simulink model "c10mimps"  (R2017a)
settings: Solver=ode45  StartTime=0.0  StopTime=10.0  RelTol=1e-10
undefined symbols (not defined in the file): n, ww
libraries: simulink x1
settings Model: Creator=Professor Dingyu Xue  LastModifiedBy=Professor Dingyu Xue
settings DataIOCC: SaveFormat=Array
settings OptimizationCC: LifeSpan=inf
settings DebuggingCC: FcnCallInpInsideContextMsg=warning  SFExecutionAtInitializationDiag=none
settings HardwareCC: ProdBitPerSizeT=32  ProdBitPerPtrDiffT=32  ProdWordSize=32  ProdHWDeviceType=Specified

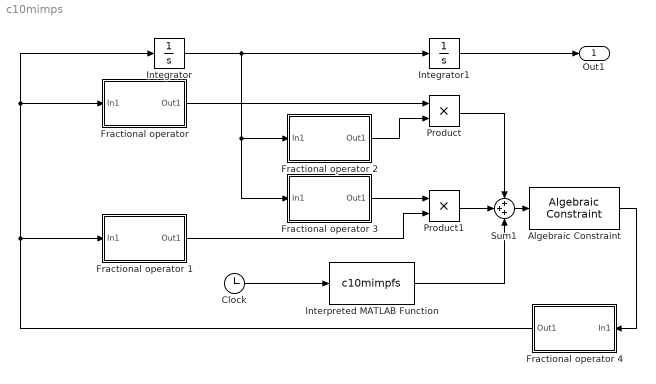
== system c10mimps ==
  Algebraic Constraint : simulink/Math Operations/Algebraic Constraint  z0=0
      settings: SourceProductName=Simulink  SourceProductBaseCode=SL
  Clock : Clock
  "Fractional operator " : Subsystem  mask{gam=-0.2, ww=ww, n=n, kF1=on, kF=Oustaloup filter}
      mask prompts: gam "Derivative order gamma"; ww "Frequency range [wb,wh]"; n "Apprixmation order"; kF1 "Is a low-pass filter required?"; kF "Filter type"
      mask init:
      | wb=ww(1); wh=ww(2); 
      | if kF==1, G=ousta_fod(gam,n,wb,wh);
      | else, G=new_fod(gam,n,wb,wh); end
      | num=G.num{1}; den=G.den{1}; T=1/wh; str='Fractional\n';
      | if isnumeric(gam)
      | 	if gam>0, str=[str, 'Der  s^' num2str(gam) ];
      | 	else, str=[str, 'Int  s^{' num2str(gam) '}']; end
      | else, str=[str, 'Der  s^gam']; end
      | if kF1==1, G=G*tf(1,[T 1]); end
      mask TypeOptions kF: Oustaloup filter | Modified Oustaloup filter
      mask Display: disp(str)
  Fractional operator 1 : Subsystem  mask{gam=-0.3, ww=ww, n=n, kF1=on, kF=Oustaloup filter}
      mask prompts: gam "Derivative order gamma"; ww "Frequency range [wb,wh]"; n "Apprixmation order"; kF1 "Is a low-pass filter required?"; kF "Filter type"
      mask init: same as c10mimps/Fractional operator 
      mask TypeOptions kF: Oustaloup filter | Modified Oustaloup filter
      mask Display: disp(str)
  Fractional operator 2 : Subsystem  mask{gam=-0.8, ww=ww, n=n, kF1=on, kF=Oustaloup filter}
      mask prompts: gam "Derivative order gamma"; ww "Frequency range [wb,wh]"; n "Apprixmation order"; kF1 "Is a low-pass filter required?"; kF "Filter type"
      mask init: same as c10mimps/Fractional operator 
      mask TypeOptions kF: Oustaloup filter | Modified Oustaloup filter
      mask Display: disp(str)
  Fractional operator 3 : Subsystem  mask{gam=-0.7, ww=ww, n=n, kF1=on, kF=Oustaloup filter}
      mask prompts: gam "Derivative order gamma"; ww "Frequency range [wb,wh]"; n "Apprixmation order"; kF1 "Is a low-pass filter required?"; kF "Filter type"
      mask init: same as c10mimps/Fractional operator 
      mask TypeOptions kF: Oustaloup filter | Modified Oustaloup filter
      mask Display: disp(str)
  Fractional operator 4 : Subsystem  mask{gam=0.2, ww=ww, n=n, kF1=on, kF=Oustaloup filter}
      mask prompts: gam "Derivative order gamma"; ww "Frequency range [wb,wh]"; n "Apprixmation order"; kF1 "Is a low-pass filter required?"; kF "Filter type"
      mask init: same as c10mimps/Fractional operator 
      mask TypeOptions kF: Oustaloup filter | Modified Oustaloup filter
      mask Display: disp(str)
  Integrator : Integrator  InitialCondition=-1/2
  Integrator1 : Integrator  InitialCondition=1
  Interpreted MATLAB Function : MATLABFcn  MATLABFcn=c10mimpfs
  Product : Product
  Product1 : Product
  Sum1 : Sum  Inputs=+++
  Out1 : Outport
  wires:
  Integrator/1 -> Integrator1/1, Fractional operator 2/1(In1), Fractional operator 3/1(In1)
  Fractional operator 4/1(Out1) -> Integrator/1, "Fractional operator "/1(In1), Fractional operator 1/1(In1)
  Fractional operator 2/1(Out1) -> Product/2
  "Fractional operator "/1(Out1) -> Product/1
  Fractional operator 3/1(Out1) -> Product1/1
  Fractional operator 1/1(Out1) -> Product1/2
  Clock/1 -> Interpreted MATLAB Function/1
  Product1/1 -> Sum1/2
  Product/1 -> Sum1/1
  Sum1/1 -> Algebraic Constraint/1
  Algebraic Constraint/1 -> Fractional operator 4/1(In1)
  Integrator1/1 -> Out1/1
  Interpreted MATLAB Function/1 -> Sum1/3

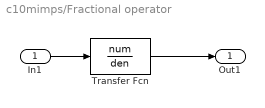
== system c10mimps/Fractional operator  ==
  In1 : Inport
  Transfer Fcn : TransferFcn  Numerator=num  Denominator=den
  Out1 : Outport
  wires:
  In1/1 -> Transfer Fcn/1
  Transfer Fcn/1 -> Out1/1

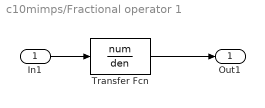
== system c10mimps/Fractional operator 1 ==
  In1 : Inport
  Transfer Fcn : TransferFcn  Numerator=num  Denominator=den
  Out1 : Outport
  wires:
  Transfer Fcn/1 -> Out1/1
  In1/1 -> Transfer Fcn/1

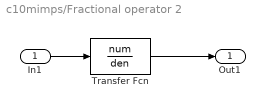
== system c10mimps/Fractional operator 2 ==
  In1 : Inport
  Transfer Fcn : TransferFcn  Numerator=num  Denominator=den
  Out1 : Outport
  wires:
  Transfer Fcn/1 -> Out1/1
  In1/1 -> Transfer Fcn/1

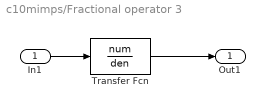
== system c10mimps/Fractional operator 3 ==
  In1 : Inport
  Transfer Fcn : TransferFcn  Numerator=num  Denominator=den
  Out1 : Outport
  wires:
  In1/1 -> Transfer Fcn/1
  Transfer Fcn/1 -> Out1/1

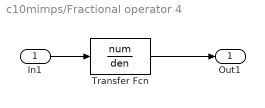
== system c10mimps/Fractional operator 4 ==
  In1 : Inport
  Transfer Fcn : TransferFcn  Numerator=num  Denominator=den
  Out1 : Outport
  wires:
  In1/1 -> Transfer Fcn/1
  Transfer Fcn/1 -> Out1/1
